simulink model "Test"  (R2023b)
settings: Solver=FixedStepDiscrete  StartTime=0.0  StopTime=inf  RelTol=1e-3
model workspace (MATLAB code in the model file):
  | cmdLim = Simulink.Parameter;
  | cmdLim.Value = 15;
  | cmdLim.Description = 'Limit for controlling the maximum surface command angle.';
  | cmdLim.Min = 0;
  | cmdLim.Max = 90;
  | cmdLim.DocUnits = 'deg';
  | 
  | dispGain = Simulink.Parameter;
  | dispGain.Value = 0.75;
  | dispGain.Description = 'Gain applied to the displacement error.';
  | dispGain.Min = 0;
  | dispGain.Max = [];
  | dispGain.DocUnits = 'deg/sec/deg';
  | 
  | dispLim = Simulink.Parameter;
  | dispLim.Value = 30;
  | dispLim.Description = 'Limit for controlling the maximum commanded angle.';
  | dispLim.Min = 0;
  | dispLim.Max = 180;
  | dispLim.DocUnits = 'deg';
  | 
  | intGain = Simulink.Parameter;
  | intGain.Value = 0.5;
  | intGain.Description = 'Gain applied to the integral error.';
  | intGain.Min = 0;
  | intGain.Max = [];
  | intGain.DocUnits = 'deg/sec/deg/sec';
  | 
  | intLim = Simulink.Parameter;
  | intLim.Value = 5;
  | intLim.Description = 'Limit for controlling the maximum commanded angle.';
  | intLim.Min = 0;
  | intLim.Max = 90;
  | intLim.DocUnits = 'deg';
  | 
  | rateGain = Simulink.Parameter;
  | rateGain.Value = 2;
  | rateGain.Description = 'Gain applied to the rate error.';
  | rateGain.Min = 0;
  | rateGain.Max = [];
  | rateGain.DocUnits = 'deg/deg/sec';
  | 
  | rateLim = Simulink.Parameter;
  | rateLim.Value = 6;
  | rateLim.Description = 'Limit for controlling the maximum commanded angle.';
  | rateLim.Min = 0;
  | rateLim.Max = 180;
  | rateLim.DocUnits = 'deg/sec';
  | 
  | hdgGain = Simulink.Parameter;
  | hdgGain.Value = 0.015;
libraries: simulink x33, arduinolib x17, hdlsllib x14, canmsglib x2
settings Model: RequirementInfo={} %GIDa_fe9045fd_0412_4b6e_8206_617cc20e6fde  DataDictionary=Time.sldd  FPTRunName=Active  ExtModeTrigDuration=2  Creator=jorda  LastModifiedBy=jorda
settings SolverCC: AlgebraicLoopSolver=TrustRegion  AutoInsertRateTranBlk=on
settings DataIOCC: SaveOutput=off  SignalLogging=off  DSMLogging=off  SaveTime=off
settings OptimizationCC: UseDivisionForNetSlopeComputation=on  GainParamInheritBuiltInType=on  UseFloatMulNetSlope=on  UseSpecifiedMinMax=on  EnhancedBackFolding=on  PassReuseOutputArgsAs=Individual arguments  ZeroExternalMemoryAtStartup=off  ZeroInternalMemoryAtStartup=off  NoFixptDivByZeroProtection=on  EfficientFloat2IntCast=on  LifeSpan=1  MaxStackSize=64  OptimizeBlockOrder=speed  DifferentSizesBufferReuse=on  OptimizationCustomize=off  EfficientTunableParamExpr=on
settings DebuggingCC: MultiTaskDSMMsg=none  UnconnectedInputMsg=warning  UnconnectedOutputMsg=warning  UnconnectedLineMsg=warning  SFUnexpectedBacktrackingDiag=warning  SFNoUnconditionalDefaultTransitionDiag=warning  SFExecutionAtInitializationDiag=none  ArithmeticOperatorsInVariantConditions=warning
settings HardwareCC: ProdBitPerInt=16  ProdBitPerPointer=16  ProdBitPerSizeT=16  ProdBitPerPtrDiffT=16  ProdLargestAtomicFloat=None  ProdWordSize=8  ProdHWDeviceType=Atmel->AVR
settings ModelReferenceCC: EnableRefExpFcnMdlSchedulingChecks=on
settings SFSimCC: MATLABDynamicMemAlloc=off
settings RTWCC: Description=Embedded Coder  SystemTargetFile=ert.tlc  HardwareBoard=Arduino Mega 2560  TemplateMakefile=ert_default_tmf  Toolchain=Arduino AVR  BuildConfiguration=Faster Runs  DLArmComputeVersion=19.05
settings CodeAppCC: ForceParamTrailComments=on  IgnoreCustomStorageClasses=off  OperatorAnnotations=on  SimulinkDataObjDesc=on  SFDataObjDesc=on  CustomSymbolStrGlobalVar=rt$N$M  CustomSymbolStrType=$N$M  CustomSymbolStrFcn=$N$M$F  CustomSymbolStrMacro=$N$M  InsertBlockDesc=on  EnableCustomComments=on  ReqsInCode=on
settings ERTTargetCC: UtilityFuncGeneration=Shared location  MultiwordLength=2048  IncludeMdlTerminateFcn=off  CombineSignalStateStructs=on  SuppressErrorStatus=on  SupportAbsoluteTime=off  SupportNonFinite=off  SupportComplex=off  SupportContinuousTime=on  SupportVariableSizeSignals=on  ExtModeTransport=3  ExtModeStaticAlloc=on  ExtModeAutomaticAllocSize=off  ExtModeStaticAllocSize=2048  ExtModeMexFile=ext_xcp  ExtModeIntrfLevel=Level2 - Open  ERTFilePackagingFormat=CompactWithDataFile
settings ConfigComp: CovScope=ReferencedModels  CovSaveName=covdata_rollAP  CovMetricSettings=dcmtrwe  CovHTMLOptions=-sRT=1 -aTS=1 -bRG=1 -bTC=1 -hTR=1 -nFC=0 -scm=1 -bcm=1 -xEv=0  CovSaveCumulativeToWorkspaceVar=on  CovSaveSingleToWorkspaceVar=on  CovCumulativeVarName=covCumulativeData_rollAP  CovReportOnPause=off  CovExternalEMLEnable=off  CovSFcnEnable=off

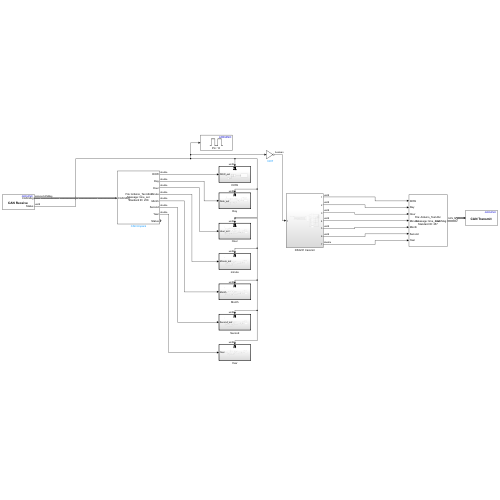
[thumbnail: Simulink's stored preview of the top-level diagram]
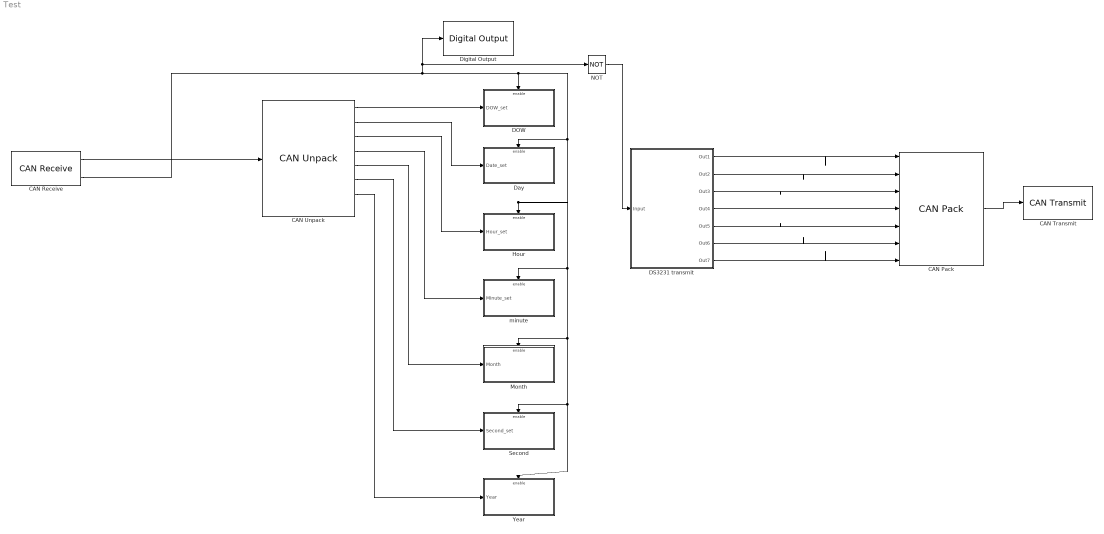
== system Test ==
  CAN Pack : canmsglib/CAN Pack  CANdbFile=C:\Users\jorda\Documents\Arduino_Test.dbc  MsgList=time_now  MsgName=time_now  MsgIDType=Standard (11-bit identifier)  MsgIdentifier=257  MsgLength=7  Remote=off  ApplyMinMax=off  BusOutput=on  SignalInfo={'DOW','37','3','LE','unsigned','Standard','0','1','0','0','7';'Day','24','5','LE','unsigned','Standard','0','1','0','0','31';'Hour','16','5','LE','unsigned','Standard','0','1','0','0','31';'Minute','8','6','LE','unsigned','Standard','0','1','0','0','63';'Month','32','4','LE','unsigned','Standard','0','1','0','0','15';'Second','0','6','LE','unsigned','Standard','0','1','0','0','63';'Year','40','12','LE','unsigned','Standard','0','1','0','0','4095'}
      settings: LibrarySourceBlock=embeddedtargetslib/Host Communication/CAN Pack  DataFormat=CANdb specified signals
  CAN Receive : arduinolib/CAN Receive  outputDataType=CAN Msg  identifierType=Standard (11-bit identifier)  messageId=100  msgLength=8  SampleTime=0.1  outputError=off  outputRemote=off
  CAN Transmit : arduinolib/CAN Transmit  inputDataType=CAN Msg  BlockingMode_=off  BlockTimeout_=1  outputStatus=off  identifierType=Standard (11-bit identifier)  messageId=102  msgLength=8  remoteFrame=off
  CAN Unpack : canmsglib/CAN Unpack  CANdbFile=C:\Users\jorda\Documents\Arduino_Test.dbc  MsgList=time_set  MsgName=time_set  MsgIDType=Standard (11-bit identifier)  MsgIdentifier=258  MsgLength=7  SignalInfo={'DOW','37','3','LE','unsigned','Standard','0','1','0','0','7';'Day','24','5','LE','unsigned','Standard','0','1','0','0','31';'Hour','16','5','LE','unsigned','Standard','0','1','0','0','31';'Minute','8','6','LE','unsigned','Standard','0','1','0','0','63';'Month','32','4','LE','unsigned','Standard','0','1','0','0','15';'Second','0','6','LE','unsigned','Standard','0','1','0','0','63';'Year','40','12','LE','unsigned','Standard','0','1','0','0','4095'}  IDPort=off  TimestampPort=off  ErrorPort=off  RemotePort=off  LengthPort=off  StatusPort=on  ApplyMinMax=off
      settings: LibrarySourceBlock=embeddedtargetslib/Host Communication/CAN Unpack  DataFormat=CANdb specified signals
  DOW : Subsystem
  DS3231 transmit : Subsystem
  Day : Subsystem
  Digital Output : arduinolib/Digital Output  pinNumber=13  Direction=output  blockPlatform=arduino
  Hour : Subsystem
  Month : Subsystem
  NOT : Logic  Operator=NOT  IconShape=distinctive  AllPortsSameDT=off  OutDataTypeStr=boolean
  Second : Subsystem
  Year : Subsystem
  minute : Subsystem
  wires:
  CAN Pack/1 -> CAN Transmit/1
  DS3231 transmit/1(Out1) -> CAN Pack/1
  DS3231 transmit/2(Out2) -> CAN Pack/2
  DS3231 transmit/3(Out3) -> CAN Pack/3
  DS3231 transmit/4(Out4) -> CAN Pack/4
  DS3231 transmit/5(Out5) -> CAN Pack/5
  DS3231 transmit/6(Out6) -> CAN Pack/6
  DS3231 transmit/7(Out7) -> CAN Pack/7
  CAN Receive/1 -> CAN Unpack/1
  CAN Receive/2 -> NOT/1, Digital Output/1, Day/Enable, Year/Enable, Second/Enable, Month/Enable, minute/Enable, Hour/Enable, DOW/Enable
  NOT/1 -> DS3231 transmit/1(Input)
  CAN Unpack/1 -> DOW/1(DOW_set)
  CAN Unpack/2 -> Day/1(Date_set)
  CAN Unpack/3 -> Hour/1(Hour_set)
  CAN Unpack/4 -> minute/1(Minute_set)
  CAN Unpack/5 -> Month/1(Month)
  CAN Unpack/6 -> Second/1(Second_set)
  CAN Unpack/7 -> Year/1(Year)

== system Test/DOW ==
  DOW_set : Inport
  Enable : EnablePort
  Bitwise AND : simulink/Logic and Bit Operations/Bitwise Operator  logicop=AND  UseBitMask=off  NumInputPorts=2  BitMask=bin2dec('11011001')  BitMaskRealWorld=Stored Integer
      settings: LibrarySourceBlock=|
      | simulink/Quick Insert/Logic and Bit
      | Operations/Bitwise AND
  Constant : Constant  Value=0x07
  Data Type Conversion : DataTypeConversion  OutDataTypeStr=uint8  SaturateOnIntegerOverflow=off  RndMeth=Floor
  I2C Write : arduinolib/I2C Write  I2CModule=0  Mode=Master  SlaveAddress=0x68  SlaveByteOrder=BigEndian  Direction=Transmitter  RegisterAddressMode=on  RegisterAddress=0x03  SlaveDataType=uint8  DataLength=1  NoAck=off  RepeatedStart=off  OutputStatus=off  blockPlatform=ARDUINO
  wires:
  Bitwise AND/1 -> I2C Write/1
  DOW_set/1 -> Data Type Conversion/1
  Constant/1 -> Bitwise AND/2
  Data Type Conversion/1 -> Bitwise AND/1

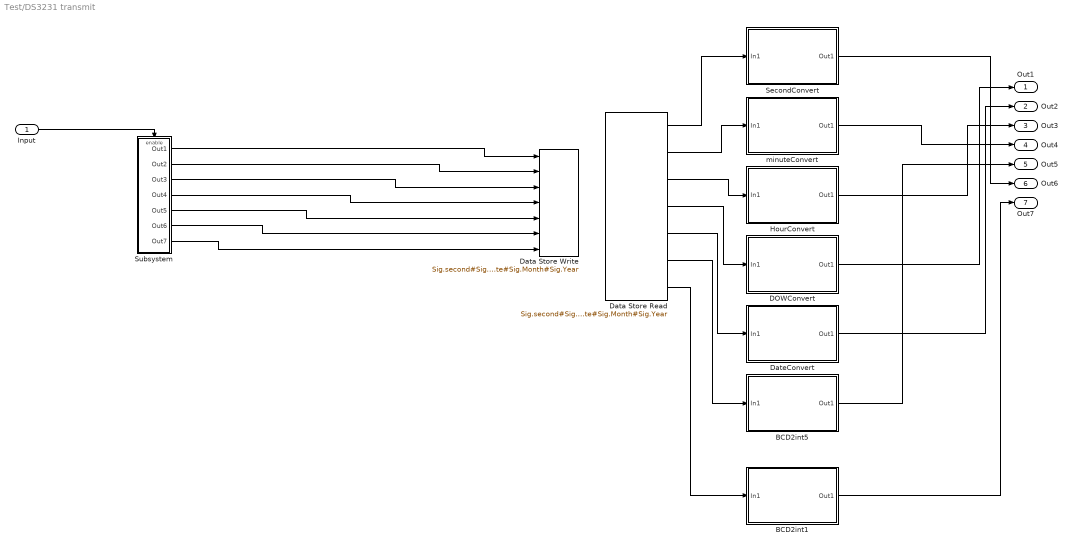
== system Test/DS3231 transmit ==
  Input : Inport
  BCD2int1 : Subsystem
  BCD2int5 : Subsystem
  DOWConvert : Subsystem
  Data Store Read : DataStoreRead  DataStoreName=Sig  DataStoreElements=Sig.second#Sig.minute#Sig.hour#Sig.DOW#Sig.Date#Sig.Month#Sig.Year  IndexOptions=Index vector (dialog)  Indices=1  OutputSizes=1
  Data Store Write : DataStoreWrite  DataStoreName=Sig  DataStoreElements=Sig.second#Sig.minute#Sig.hour#Sig.DOW#Sig.Date#Sig.Month#Sig.Year  IndexOptions=Index vector (dialog)  Indices=1  OutputSizes=1
  DateConvert : Subsystem
  HourConvert : Subsystem
  SecondConvert : Subsystem
  Subsystem : Subsystem
  minuteConvert : Subsystem
  Out1 : Outport
  Out2 : Outport  Port=2
  Out3 : Outport  Port=3
  Out4 : Outport  Port=4
  Out5 : Outport  Port=5
  Out6 : Outport  Port=6
  Out7 : Outport  Port=7
  wires:
  Data Store Read/6 -> BCD2int5/1(In1)
  Data Store Read/3 -> HourConvert/1(In1)
  Data Store Read/1 -> SecondConvert/1(In1)
  SecondConvert/1(Out1) -> Out6/1
  Data Store Read/7 -> BCD2int1/1(In1)
  Data Store Read/2 -> minuteConvert/1(In1)
  Data Store Read/4 -> DOWConvert/1(In1)
  Data Store Read/5 -> DateConvert/1(In1)
  HourConvert/1(Out1) -> Out3/1
  DateConvert/1(Out1) -> Out2/1
  DOWConvert/1(Out1) -> Out1/1
  BCD2int5/1(Out1) -> Out5/1
  minuteConvert/1(Out1) -> Out4/1
  BCD2int1/1(Out1) -> Out7/1
  Subsystem/1(Out1) -> Data Store Write/1
  Subsystem/2(Out2) -> Data Store Write/2
  Subsystem/3(Out3) -> Data Store Write/3
  Subsystem/4(Out4) -> Data Store Write/4
  Subsystem/5(Out5) -> Data Store Write/5
  Subsystem/6(Out6) -> Data Store Write/6
  Subsystem/7(Out7) -> Data Store Write/7
  Input/1 -> Subsystem/Enable

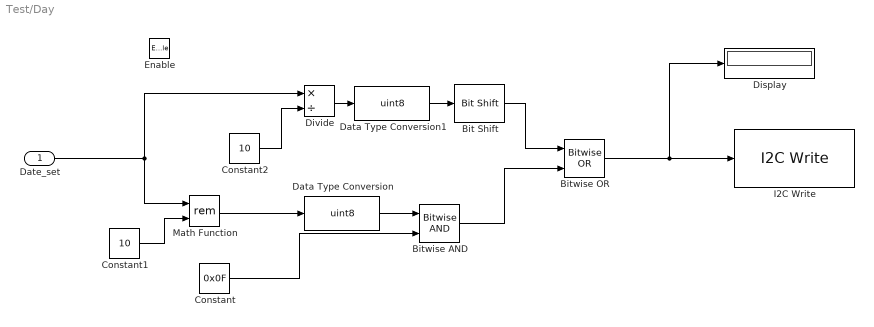
== system Test/Day ==
  Date_set : Inport
  Enable : EnablePort
  Bit Shift : hdlsllib/Logic and Bit Operations/Bit Shift  mode=Shift Left Logical  N=4
  Bitwise AND : simulink/Logic and Bit Operations/Bitwise Operator  logicop=AND  UseBitMask=off  NumInputPorts=2  BitMask=bin2dec('11011001')  BitMaskRealWorld=Stored Integer
      settings: LibrarySourceBlock=|
      | simulink/Quick Insert/Logic and Bit
      | Operations/Bitwise AND
  Bitwise OR : simulink/Logic and Bit Operations/Bitwise Operator  logicop=OR  UseBitMask=off  NumInputPorts=2  BitMask=bin2dec('11011001')  BitMaskRealWorld=Stored Integer
      settings: LibrarySourceBlock=|
      | simulink/Quick Insert/Logic and Bit
      | Operations/Bitwise OR
  Constant : Constant  Value=0x0F
  Constant1 : Constant  Value=10
  Constant2 : Constant  Value=10
  Data Type Conversion : DataTypeConversion  OutDataTypeStr=uint8  SaturateOnIntegerOverflow=off  RndMeth=Floor
  Data Type Conversion1 : DataTypeConversion  OutDataTypeStr=uint8  SaturateOnIntegerOverflow=off  RndMeth=Floor
  Display : Display
      settings: Format=hex (Stored Integer)
  Divide : Product  Inputs=*/
  I2C Write : arduinolib/I2C Write  I2CModule=0  Mode=Master  SlaveAddress=0x68  SlaveByteOrder=BigEndian  Direction=Transmitter  RegisterAddressMode=on  RegisterAddress=0x04  SlaveDataType=uint8  DataLength=1  NoAck=off  RepeatedStart=off  OutputStatus=off  blockPlatform=ARDUINO
  Math Function : Math  Operator=rem
  wires:
  Constant/1 -> Bitwise AND/2
  Constant2/1 -> Divide/2
  Bit Shift/1 -> Bitwise OR/1
  Bitwise AND/1 -> Bitwise OR/2
  Data Type Conversion1/1 -> Bit Shift/1
  Divide/1 -> Data Type Conversion1/1
  Bitwise OR/1 -> Display/1, I2C Write/1
  Data Type Conversion/1 -> Bitwise AND/1
  Constant1/1 -> Math Function/2
  Math Function/1 -> Data Type Conversion/1
  Date_set/1 -> Math Function/1, Divide/1

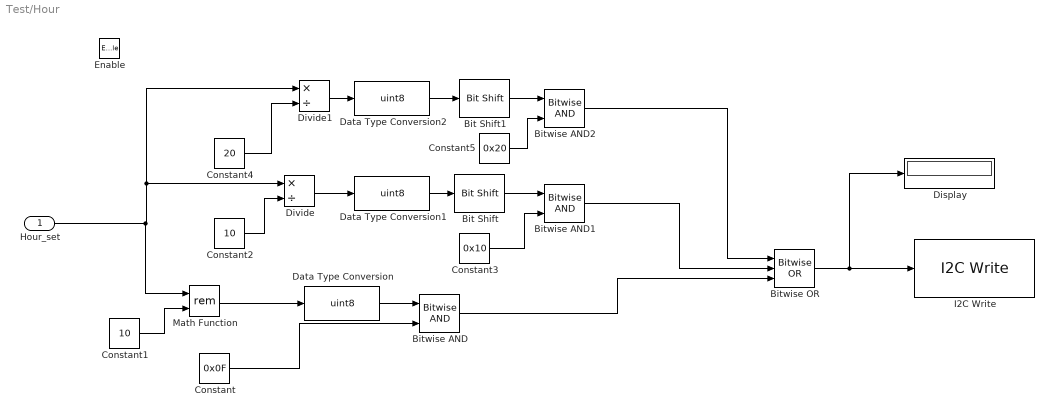
== system Test/Hour ==
  Hour_set : Inport
  Enable : EnablePort
  Bit Shift : hdlsllib/Logic and Bit Operations/Bit Shift  mode=Shift Left Logical  N=4
  Bit Shift1 : hdlsllib/Logic and Bit Operations/Bit Shift  mode=Shift Left Logical  N=5
  Bitwise AND : simulink/Logic and Bit Operations/Bitwise Operator  logicop=AND  UseBitMask=off  NumInputPorts=2  BitMask=bin2dec('11011001')  BitMaskRealWorld=Stored Integer
      settings: LibrarySourceBlock=|
      | simulink/Quick Insert/Logic and Bit
      | Operations/Bitwise AND
  Bitwise AND1 : simulink/Logic and Bit Operations/Bitwise Operator  logicop=AND  UseBitMask=off  NumInputPorts=2  BitMask=bin2dec('11011001')  BitMaskRealWorld=Stored Integer
      settings: LibrarySourceBlock=|
      | simulink/Quick Insert/Logic and Bit
      | Operations/Bitwise AND
  Bitwise AND2 : simulink/Logic and Bit Operations/Bitwise Operator  logicop=AND  UseBitMask=off  NumInputPorts=2  BitMask=bin2dec('11011001')  BitMaskRealWorld=Stored Integer
      settings: LibrarySourceBlock=|
      | simulink/Quick Insert/Logic and Bit
      | Operations/Bitwise AND
  Bitwise OR : simulink/Logic and Bit Operations/Bitwise Operator  logicop=OR  UseBitMask=off  NumInputPorts=3  BitMask=bin2dec('11011001')  BitMaskRealWorld=Stored Integer
      settings: LibrarySourceBlock=|
      | simulink/Quick Insert/Logic and Bit
      | Operations/Bitwise OR
  Constant : Constant  Value=0x0F
  Constant1 : Constant  Value=10
  Constant2 : Constant  Value=10
  Constant3 : Constant  Value=0x10
  Constant4 : Constant  Value=20
  Constant5 : Constant  Value=0x20
  Data Type Conversion : DataTypeConversion  OutDataTypeStr=uint8  SaturateOnIntegerOverflow=off  RndMeth=Floor
  Data Type Conversion1 : DataTypeConversion  OutDataTypeStr=uint8  SaturateOnIntegerOverflow=off  RndMeth=Floor
  Data Type Conversion2 : DataTypeConversion  OutDataTypeStr=uint8  SaturateOnIntegerOverflow=off  RndMeth=Floor
  Display : Display
      settings: Format=hex (Stored Integer)
  Divide : Product  Inputs=*/
  Divide1 : Product  Inputs=*/
  I2C Write : arduinolib/I2C Write  I2CModule=0  Mode=Master  SlaveAddress=0x68  SlaveByteOrder=BigEndian  Direction=Transmitter  RegisterAddressMode=on  RegisterAddress=0x02  SlaveDataType=uint8  DataLength=1  NoAck=off  RepeatedStart=off  OutputStatus=off  blockPlatform=ARDUINO
  Math Function : Math  Operator=rem
  wires:
  Constant/1 -> Bitwise AND/2
  Constant2/1 -> Divide/2
  Bitwise AND/1 -> Bitwise OR/3
  Data Type Conversion1/1 -> Bit Shift/1
  Divide/1 -> Data Type Conversion1/1
  Bitwise OR/1 -> Display/1, I2C Write/1
  Data Type Conversion/1 -> Bitwise AND/1
  Constant1/1 -> Math Function/2
  Math Function/1 -> Data Type Conversion/1
  Bit Shift/1 -> Bitwise AND1/1
  Constant3/1 -> Bitwise AND1/2
  Bitwise AND1/1 -> Bitwise OR/2
  Divide1/1 -> Data Type Conversion2/1
  Constant4/1 -> Divide1/2
  Data Type Conversion2/1 -> Bit Shift1/1
  Bit Shift1/1 -> Bitwise AND2/1
  Constant5/1 -> Bitwise AND2/2
  Bitwise AND2/1 -> Bitwise OR/1
  Hour_set/1 -> Math Function/1, Divide/1, Divide1/1

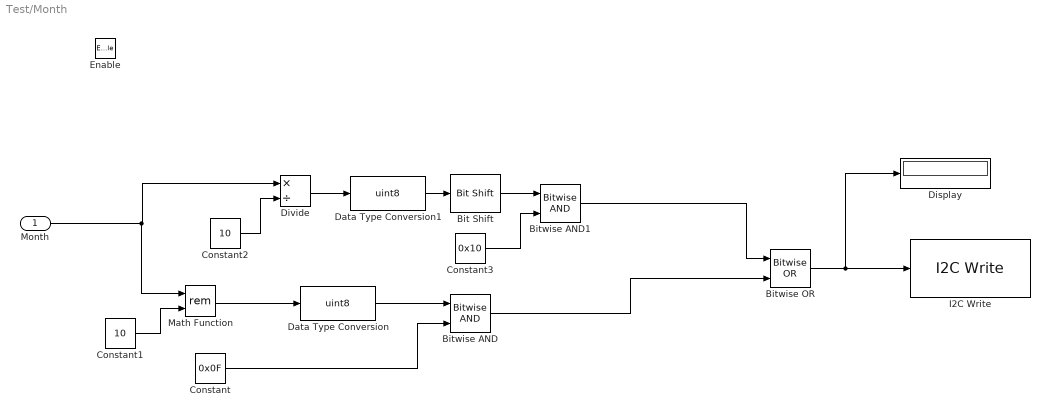
== system Test/Month ==
  Month : Inport
  Enable : EnablePort
  Bit Shift : hdlsllib/Logic and Bit Operations/Bit Shift  mode=Shift Left Logical  N=4
  Bitwise AND : simulink/Logic and Bit Operations/Bitwise Operator  logicop=AND  UseBitMask=off  NumInputPorts=2  BitMask=bin2dec('11011001')  BitMaskRealWorld=Stored Integer
      settings: LibrarySourceBlock=|
      | simulink/Quick Insert/Logic and Bit
      | Operations/Bitwise AND
  Bitwise AND1 : simulink/Logic and Bit Operations/Bitwise Operator  logicop=AND  UseBitMask=off  NumInputPorts=2  BitMask=bin2dec('11011001')  BitMaskRealWorld=Stored Integer
      settings: LibrarySourceBlock=|
      | simulink/Quick Insert/Logic and Bit
      | Operations/Bitwise AND
  Bitwise OR : simulink/Logic and Bit Operations/Bitwise Operator  logicop=OR  UseBitMask=off  NumInputPorts=2  BitMask=bin2dec('11011001')  BitMaskRealWorld=Stored Integer
      settings: LibrarySourceBlock=|
      | simulink/Quick Insert/Logic and Bit
      | Operations/Bitwise OR
  Constant : Constant  Value=0x0F
  Constant1 : Constant  Value=10
  Constant2 : Constant  Value=10
  Constant3 : Constant  Value=0x10
  Data Type Conversion : DataTypeConversion  OutDataTypeStr=uint8  SaturateOnIntegerOverflow=off  RndMeth=Floor
  Data Type Conversion1 : DataTypeConversion  OutDataTypeStr=uint8  SaturateOnIntegerOverflow=off  RndMeth=Floor
  Display : Display
      settings: Format=hex (Stored Integer)
  Divide : Product  Inputs=*/
  I2C Write : arduinolib/I2C Write  I2CModule=0  Mode=Master  SlaveAddress=0x68  SlaveByteOrder=BigEndian  Direction=Transmitter  RegisterAddressMode=on  RegisterAddress=0x05  SlaveDataType=uint8  DataLength=1  NoAck=off  RepeatedStart=off  OutputStatus=off  blockPlatform=ARDUINO
  Math Function : Math  Operator=rem
  wires:
  Constant/1 -> Bitwise AND/2
  Constant2/1 -> Divide/2
  Bitwise AND/1 -> Bitwise OR/2
  Data Type Conversion1/1 -> Bit Shift/1
  Divide/1 -> Data Type Conversion1/1
  Bitwise OR/1 -> Display/1, I2C Write/1
  Data Type Conversion/1 -> Bitwise AND/1
  Constant1/1 -> Math Function/2
  Math Function/1 -> Data Type Conversion/1
  Bit Shift/1 -> Bitwise AND1/1
  Constant3/1 -> Bitwise AND1/2
  Bitwise AND1/1 -> Bitwise OR/1
  Month/1 -> Math Function/1, Divide/1

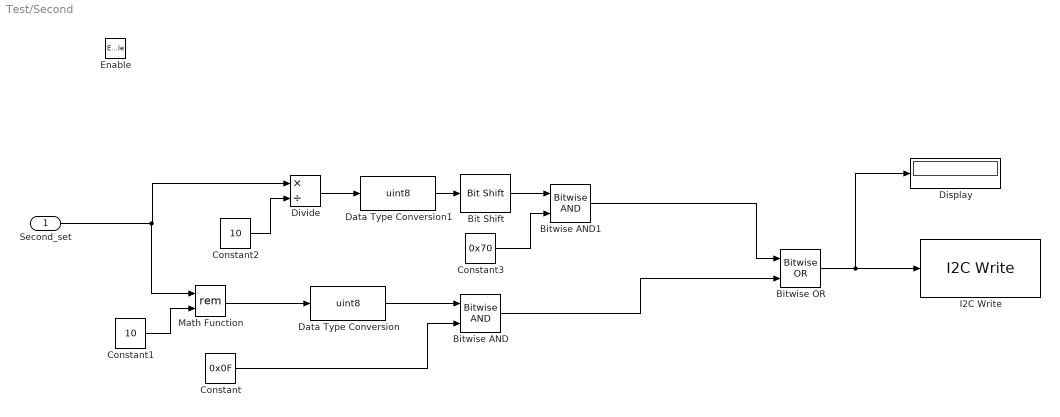
== system Test/Second ==
  Second_set : Inport
  Enable : EnablePort
  Bit Shift : hdlsllib/Logic and Bit Operations/Bit Shift  mode=Shift Left Logical  N=4
  Bitwise AND : simulink/Logic and Bit Operations/Bitwise Operator  logicop=AND  UseBitMask=off  NumInputPorts=2  BitMask=bin2dec('11011001')  BitMaskRealWorld=Stored Integer
      settings: LibrarySourceBlock=|
      | simulink/Quick Insert/Logic and Bit
      | Operations/Bitwise AND
  Bitwise AND1 : simulink/Logic and Bit Operations/Bitwise Operator  logicop=AND  UseBitMask=off  NumInputPorts=2  BitMask=bin2dec('11011001')  BitMaskRealWorld=Stored Integer
      settings: LibrarySourceBlock=|
      | simulink/Quick Insert/Logic and Bit
      | Operations/Bitwise AND
  Bitwise OR : simulink/Logic and Bit Operations/Bitwise Operator  logicop=OR  UseBitMask=off  NumInputPorts=2  BitMask=bin2dec('11011001')  BitMaskRealWorld=Stored Integer
      settings: LibrarySourceBlock=|
      | simulink/Quick Insert/Logic and Bit
      | Operations/Bitwise OR
  Constant : Constant  Value=0x0F
  Constant1 : Constant  Value=10
  Constant2 : Constant  Value=10
  Constant3 : Constant  Value=0x70
  Data Type Conversion : DataTypeConversion  OutDataTypeStr=uint8  SaturateOnIntegerOverflow=off  RndMeth=Floor
  Data Type Conversion1 : DataTypeConversion  OutDataTypeStr=uint8  SaturateOnIntegerOverflow=off  RndMeth=Floor
  Display : Display
      settings: Format=hex (Stored Integer)
  Divide : Product  Inputs=*/
  I2C Write : arduinolib/I2C Write  I2CModule=0  Mode=Master  SlaveAddress=0x68  SlaveByteOrder=BigEndian  Direction=Transmitter  RegisterAddressMode=on  RegisterAddress=0x00  SlaveDataType=uint8  DataLength=1  NoAck=off  RepeatedStart=off  OutputStatus=off  blockPlatform=ARDUINO
  Math Function : Math  Operator=rem
  wires:
  Constant/1 -> Bitwise AND/2
  Constant2/1 -> Divide/2
  Bitwise AND/1 -> Bitwise OR/2
  Data Type Conversion1/1 -> Bit Shift/1
  Divide/1 -> Data Type Conversion1/1
  Bitwise OR/1 -> Display/1, I2C Write/1
  Data Type Conversion/1 -> Bitwise AND/1
  Constant1/1 -> Math Function/2
  Math Function/1 -> Data Type Conversion/1
  Bit Shift/1 -> Bitwise AND1/1
  Constant3/1 -> Bitwise AND1/2
  Bitwise AND1/1 -> Bitwise OR/1
  Second_set/1 -> Math Function/1, Divide/1

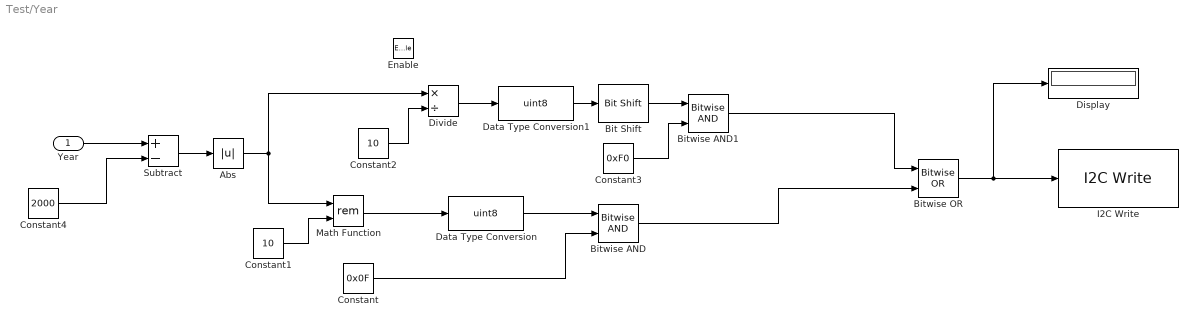
== system Test/Year ==
  Year : Inport
  Enable : EnablePort
  Abs : Abs  SaturateOnIntegerOverflow=off
  Bit Shift : hdlsllib/Logic and Bit Operations/Bit Shift  mode=Shift Left Logical  N=4
  Bitwise AND : simulink/Logic and Bit Operations/Bitwise Operator  logicop=AND  UseBitMask=off  NumInputPorts=2  BitMask=bin2dec('11011001')  BitMaskRealWorld=Stored Integer
      settings: LibrarySourceBlock=|
      | simulink/Quick Insert/Logic and Bit
      | Operations/Bitwise AND
  Bitwise AND1 : simulink/Logic and Bit Operations/Bitwise Operator  logicop=AND  UseBitMask=off  NumInputPorts=2  BitMask=bin2dec('11011001')  BitMaskRealWorld=Stored Integer
      settings: LibrarySourceBlock=|
      | simulink/Quick Insert/Logic and Bit
      | Operations/Bitwise AND
  Bitwise OR : simulink/Logic and Bit Operations/Bitwise Operator  logicop=OR  UseBitMask=off  NumInputPorts=2  BitMask=bin2dec('11011001')  BitMaskRealWorld=Stored Integer
      settings: LibrarySourceBlock=|
      | simulink/Quick Insert/Logic and Bit
      | Operations/Bitwise OR
  Constant : Constant  Value=0x0F
  Constant1 : Constant  Value=10
  Constant2 : Constant  Value=10
  Constant3 : Constant  Value=0xF0
  Constant4 : Constant  Value=2000
  Data Type Conversion : DataTypeConversion  OutDataTypeStr=uint8  SaturateOnIntegerOverflow=off  RndMeth=Floor
  Data Type Conversion1 : DataTypeConversion  OutDataTypeStr=uint8  SaturateOnIntegerOverflow=off  RndMeth=Floor
  Display : Display
      settings: Format=hex (Stored Integer)
  Divide : Product  Inputs=*/
  I2C Write : arduinolib/I2C Write  I2CModule=0  Mode=Master  SlaveAddress=0x68  SlaveByteOrder=BigEndian  Direction=Transmitter  RegisterAddressMode=on  RegisterAddress=0x06  SlaveDataType=uint8  DataLength=1  NoAck=off  RepeatedStart=off  OutputStatus=off  blockPlatform=ARDUINO
  Math Function : Math  Operator=rem
  Subtract : Sum  Inputs=+-
  wires:
  Constant/1 -> Bitwise AND/2
  Constant2/1 -> Divide/2
  Bitwise AND/1 -> Bitwise OR/2
  Data Type Conversion1/1 -> Bit Shift/1
  Divide/1 -> Data Type Conversion1/1
  Bitwise OR/1 -> Display/1, I2C Write/1
  Data Type Conversion/1 -> Bitwise AND/1
  Constant1/1 -> Math Function/2
  Math Function/1 -> Data Type Conversion/1
  Bit Shift/1 -> Bitwise AND1/1
  Constant3/1 -> Bitwise AND1/2
  Bitwise AND1/1 -> Bitwise OR/1
  Constant4/1 -> Subtract/2
  Subtract/1 -> Abs/1
  Year/1 -> Subtract/1
  Abs/1 -> Math Function/1, Divide/1

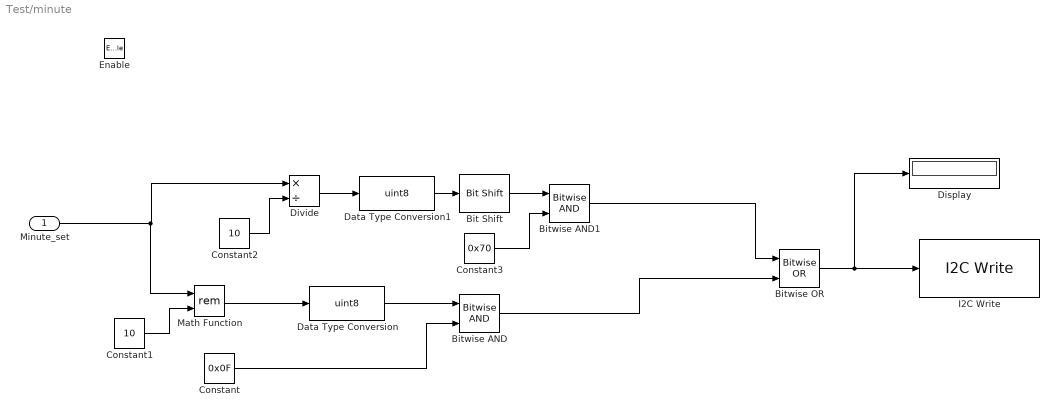
== system Test/minute ==
  Minute_set : Inport
  Enable : EnablePort
  Bit Shift : hdlsllib/Logic and Bit Operations/Bit Shift  mode=Shift Left Logical  N=4
  Bitwise AND : simulink/Logic and Bit Operations/Bitwise Operator  logicop=AND  UseBitMask=off  NumInputPorts=2  BitMask=bin2dec('11011001')  BitMaskRealWorld=Stored Integer
      settings: LibrarySourceBlock=|
      | simulink/Quick Insert/Logic and Bit
      | Operations/Bitwise AND
  Bitwise AND1 : simulink/Logic and Bit Operations/Bitwise Operator  logicop=AND  UseBitMask=off  NumInputPorts=2  BitMask=bin2dec('11011001')  BitMaskRealWorld=Stored Integer
      settings: LibrarySourceBlock=|
      | simulink/Quick Insert/Logic and Bit
      | Operations/Bitwise AND
  Bitwise OR : simulink/Logic and Bit Operations/Bitwise Operator  logicop=OR  UseBitMask=off  NumInputPorts=2  BitMask=bin2dec('11011001')  BitMaskRealWorld=Stored Integer
      settings: LibrarySourceBlock=|
      | simulink/Quick Insert/Logic and Bit
      | Operations/Bitwise OR
  Constant : Constant  Value=0x0F
  Constant1 : Constant  Value=10
  Constant2 : Constant  Value=10
  Constant3 : Constant  Value=0x70
  Data Type Conversion : DataTypeConversion  OutDataTypeStr=uint8  SaturateOnIntegerOverflow=off  RndMeth=Floor
  Data Type Conversion1 : DataTypeConversion  OutDataTypeStr=uint8  SaturateOnIntegerOverflow=off  RndMeth=Floor
  Display : Display
      settings: Format=hex (Stored Integer)
  Divide : Product  Inputs=*/
  I2C Write : arduinolib/I2C Write  I2CModule=0  Mode=Master  SlaveAddress=0x68  SlaveByteOrder=BigEndian  Direction=Transmitter  RegisterAddressMode=on  RegisterAddress=0x01  SlaveDataType=uint8  DataLength=1  NoAck=off  RepeatedStart=off  OutputStatus=off  blockPlatform=ARDUINO
  Math Function : Math  Operator=rem
  wires:
  Constant/1 -> Bitwise AND/2
  Constant2/1 -> Divide/2
  Bitwise AND/1 -> Bitwise OR/2
  Data Type Conversion1/1 -> Bit Shift/1
  Divide/1 -> Data Type Conversion1/1
  Bitwise OR/1 -> Display/1, I2C Write/1
  Data Type Conversion/1 -> Bitwise AND/1
  Constant1/1 -> Math Function/2
  Math Function/1 -> Data Type Conversion/1
  Bit Shift/1 -> Bitwise AND1/1
  Constant3/1 -> Bitwise AND1/2
  Bitwise AND1/1 -> Bitwise OR/1
  Minute_set/1 -> Math Function/1, Divide/1

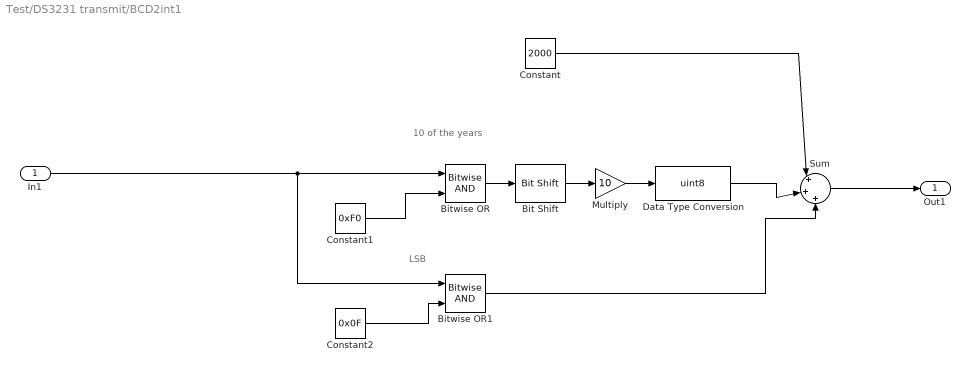
== system Test/DS3231 transmit/BCD2int1 ==
  note: LSB
  note: 10 of the years
  In1 : Inport
  Bit Shift : hdlsllib/Logic and Bit Operations/Bit Shift  mode=Shift Right Logical  N=4
  Bitwise OR : simulink/Logic and Bit Operations/Bitwise Operator  logicop=AND  UseBitMask=off  NumInputPorts=2  BitMask=bin2dec('0000FFFF')  BitMaskRealWorld=Stored Integer
      settings: LibrarySourceBlock=|
      | simulink/Quick Insert/Logic and Bit
      | Operations/Bitwise OR
  Bitwise OR1 : simulink/Logic and Bit Operations/Bitwise Operator  logicop=AND  UseBitMask=off  NumInputPorts=2  BitMask=bin2dec('0000FFFF')  BitMaskRealWorld=Stored Integer
      settings: LibrarySourceBlock=|
      | simulink/Quick Insert/Logic and Bit
      | Operations/Bitwise OR
  Constant : Constant  Value=2000
  Constant1 : Constant  Value=0xF0
  Constant2 : Constant  Value=0x0F
  Data Type Conversion : DataTypeConversion  OutDataTypeStr=uint8  SaturateOnIntegerOverflow=off  RndMeth=Floor
  Multiply : Gain  Gain=10  ParamDataTypeStr=Inherit: Same as input  LockScale=on
  Sum : Sum  Inputs=|+|+|+
  Out1 : Outport
  wires:
  Bitwise OR1/1 -> Sum/3
  Constant1/1 -> Bitwise OR/2
  Bit Shift/1 -> Multiply/1
  Bitwise OR/1 -> Bit Shift/1
  Data Type Conversion/1 -> Sum/2
  Multiply/1 -> Data Type Conversion/1
  Constant2/1 -> Bitwise OR1/2
  Sum/1 -> Out1/1
  In1/1 -> Bitwise OR1/1, Bitwise OR/1
  Constant/1 -> Sum/1

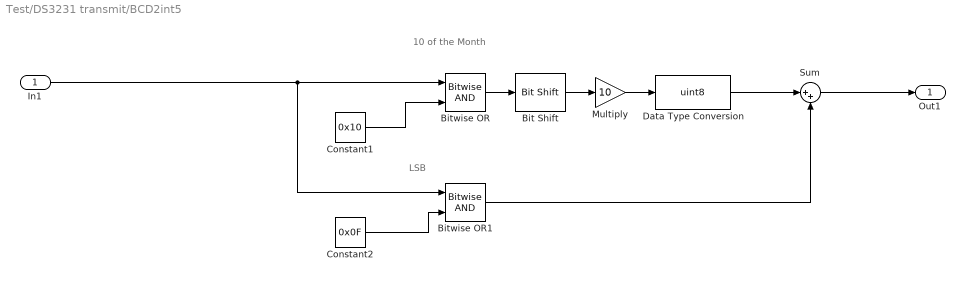
== system Test/DS3231 transmit/BCD2int5 ==
  note: LSB
  note: 10 of the Month
  In1 : Inport
  Bit Shift : hdlsllib/Logic and Bit Operations/Bit Shift  mode=Shift Right Logical  N=4
  Bitwise OR : simulink/Logic and Bit Operations/Bitwise Operator  logicop=AND  UseBitMask=off  NumInputPorts=2  BitMask=bin2dec('0000FFFF')  BitMaskRealWorld=Stored Integer
      settings: LibrarySourceBlock=|
      | simulink/Quick Insert/Logic and Bit
      | Operations/Bitwise OR
  Bitwise OR1 : simulink/Logic and Bit Operations/Bitwise Operator  logicop=AND  UseBitMask=off  NumInputPorts=2  BitMask=bin2dec('0000FFFF')  BitMaskRealWorld=Stored Integer
      settings: LibrarySourceBlock=|
      | simulink/Quick Insert/Logic and Bit
      | Operations/Bitwise OR
  Constant1 : Constant  Value=0x10
  Constant2 : Constant  Value=0x0F
  Data Type Conversion : DataTypeConversion  OutDataTypeStr=uint8  SaturateOnIntegerOverflow=off  RndMeth=Floor
  Multiply : Gain  Gain=10  ParamDataTypeStr=Inherit: Same as input  LockScale=on
  Sum : Sum  Inputs=|++
  Out1 : Outport
  wires:
  Bitwise OR1/1 -> Sum/2
  Constant1/1 -> Bitwise OR/2
  Bit Shift/1 -> Multiply/1
  Bitwise OR/1 -> Bit Shift/1
  Data Type Conversion/1 -> Sum/1
  Multiply/1 -> Data Type Conversion/1
  Constant2/1 -> Bitwise OR1/2
  Sum/1 -> Out1/1
  In1/1 -> Bitwise OR1/1, Bitwise OR/1

== system Test/DS3231 transmit/DOWConvert ==
  In1 : Inport
  Bitwise OR1 : simulink/Logic and Bit Operations/Bitwise Operator  logicop=AND  UseBitMask=off  NumInputPorts=2  BitMask=bin2dec('0000FFFF')  BitMaskRealWorld=Stored Integer
      settings: LibrarySourceBlock=|
      | simulink/Quick Insert/Logic and Bit
      | Operations/Bitwise OR
  Constant2 : Constant  Value=0x0F
  Out1 : Outport
  wires:
  Constant2/1 -> Bitwise OR1/2
  Bitwise OR1/1 -> Out1/1
  In1/1 -> Bitwise OR1/1

== system Test/DS3231 transmit/DateConvert ==
  note: LSB
  note: The 10th of Date
  In1 : Inport
  Bit Shift : hdlsllib/Logic and Bit Operations/Bit Shift  mode=Shift Right Logical  N=4
  Bitwise OR : simulink/Logic and Bit Operations/Bitwise Operator  logicop=AND  UseBitMask=off  NumInputPorts=2  BitMask=bin2dec('0000FFFF')  BitMaskRealWorld=Stored Integer
      settings: LibrarySourceBlock=|
      | simulink/Quick Insert/Logic and Bit
      | Operations/Bitwise OR
  Bitwise OR1 : simulink/Logic and Bit Operations/Bitwise Operator  logicop=AND  UseBitMask=off  NumInputPorts=2  BitMask=bin2dec('0000FFFF')  BitMaskRealWorld=Stored Integer
      settings: LibrarySourceBlock=|
      | simulink/Quick Insert/Logic and Bit
      | Operations/Bitwise OR
  Constant1 : Constant  Value=0x30
  Constant2 : Constant  Value=0x0F
  Data Type Conversion : DataTypeConversion  OutDataTypeStr=uint8  SaturateOnIntegerOverflow=off  RndMeth=Floor
  Multiply : Gain  Gain=10  ParamDataTypeStr=Inherit: Same as input  LockScale=on
  Sum : Sum  Inputs=|++
  Out1 : Outport
  wires:
  Bitwise OR1/1 -> Sum/2
  Constant1/1 -> Bitwise OR/2
  Bit Shift/1 -> Multiply/1
  Bitwise OR/1 -> Bit Shift/1
  Data Type Conversion/1 -> Sum/1
  Multiply/1 -> Data Type Conversion/1
  Constant2/1 -> Bitwise OR1/2
  Sum/1 -> Out1/1
  In1/1 -> Bitwise OR1/1, Bitwise OR/1

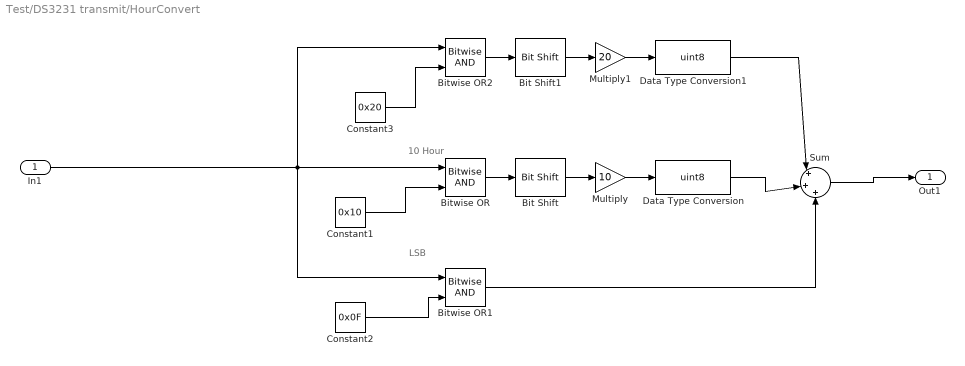
== system Test/DS3231 transmit/HourConvert ==
  note: LSB
  note: 10 Hour
  In1 : Inport
  Bit Shift : hdlsllib/Logic and Bit Operations/Bit Shift  mode=Shift Right Logical  N=4
  Bit Shift1 : hdlsllib/Logic and Bit Operations/Bit Shift  mode=Shift Right Logical  N=5
  Bitwise OR : simulink/Logic and Bit Operations/Bitwise Operator  logicop=AND  UseBitMask=off  NumInputPorts=2  BitMask=bin2dec('0000FFFF')  BitMaskRealWorld=Stored Integer
      settings: LibrarySourceBlock=|
      | simulink/Quick Insert/Logic and Bit
      | Operations/Bitwise OR
  Bitwise OR1 : simulink/Logic and Bit Operations/Bitwise Operator  logicop=AND  UseBitMask=off  NumInputPorts=2  BitMask=bin2dec('0000FFFF')  BitMaskRealWorld=Stored Integer
      settings: LibrarySourceBlock=|
      | simulink/Quick Insert/Logic and Bit
      | Operations/Bitwise OR
  Bitwise OR2 : simulink/Logic and Bit Operations/Bitwise Operator  logicop=AND  UseBitMask=off  NumInputPorts=2  BitMask=bin2dec('0000FFFF')  BitMaskRealWorld=Stored Integer
      settings: LibrarySourceBlock=|
      | simulink/Quick Insert/Logic and Bit
      | Operations/Bitwise OR
  Constant1 : Constant  Value=0x10
  Constant2 : Constant  Value=0x0F
  Constant3 : Constant  Value=0x20
  Data Type Conversion : DataTypeConversion  OutDataTypeStr=uint8  SaturateOnIntegerOverflow=off  RndMeth=Floor
  Data Type Conversion1 : DataTypeConversion  OutDataTypeStr=uint8  SaturateOnIntegerOverflow=off  RndMeth=Floor
  Multiply : Gain  Gain=10  ParamDataTypeStr=Inherit: Same as input  LockScale=on
  Multiply1 : Gain  Gain=20  ParamDataTypeStr=Inherit: Same as input  LockScale=on
  Sum : Sum  Inputs=|+|+|+
  Out1 : Outport
  wires:
  Constant1/1 -> Bitwise OR/2
  Bit Shift/1 -> Multiply/1
  Bitwise OR/1 -> Bit Shift/1
  Multiply/1 -> Data Type Conversion/1
  Constant2/1 -> Bitwise OR1/2
  Sum/1 -> Out1/1
  In1/1 -> Bitwise OR2/1, Bitwise OR1/1, Bitwise OR/1
  Bitwise OR2/1 -> Bit Shift1/1
  Bit Shift1/1 -> Multiply1/1
  Multiply1/1 -> Data Type Conversion1/1
  Bitwise OR1/1 -> Sum/3
  Data Type Conversion/1 -> Sum/2
  Data Type Conversion1/1 -> Sum/1
  Constant3/1 -> Bitwise OR2/2

== system Test/DS3231 transmit/SecondConvert ==
  note: LSB
  note: MSB
  In1 : Inport
  Bit Shift : hdlsllib/Logic and Bit Operations/Bit Shift  mode=Shift Right Logical  N=4
  Bitwise OR : simulink/Logic and Bit Operations/Bitwise Operator  logicop=AND  UseBitMask=off  NumInputPorts=2  BitMask=bin2dec('0000FFFF')  BitMaskRealWorld=Stored Integer
      settings: LibrarySourceBlock=|
      | simulink/Quick Insert/Logic and Bit
      | Operations/Bitwise OR
  Bitwise OR1 : simulink/Logic and Bit Operations/Bitwise Operator  logicop=AND  UseBitMask=off  NumInputPorts=2  BitMask=bin2dec('0000FFFF')  BitMaskRealWorld=Stored Integer
      settings: LibrarySourceBlock=|
      | simulink/Quick Insert/Logic and Bit
      | Operations/Bitwise OR
  Constant1 : Constant  Value=0xF0
  Constant2 : Constant  Value=0x0F
  Data Type Conversion : DataTypeConversion  OutDataTypeStr=uint8  SaturateOnIntegerOverflow=off  RndMeth=Floor
  Multiply : Gain  Gain=10  ParamDataTypeStr=Inherit: Same as input  LockScale=on
  Sum : Sum  Inputs=|++
  Out1 : Outport
  wires:
  Bitwise OR1/1 -> Sum/2
  Constant1/1 -> Bitwise OR/2
  Bit Shift/1 -> Multiply/1
  Bitwise OR/1 -> Bit Shift/1
  Data Type Conversion/1 -> Sum/1
  Multiply/1 -> Data Type Conversion/1
  Constant2/1 -> Bitwise OR1/2
  Sum/1 -> Out1/1
  In1/1 -> Bitwise OR1/1, Bitwise OR/1

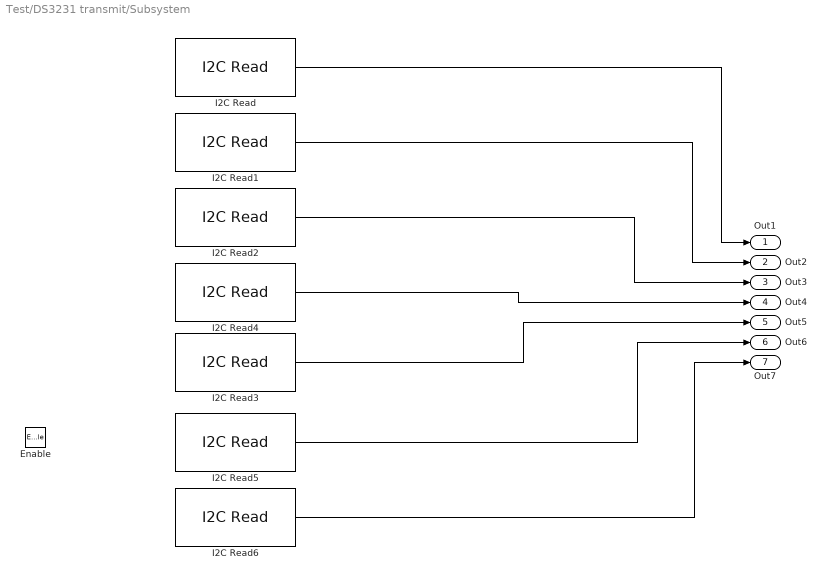
== system Test/DS3231 transmit/Subsystem ==
  Enable : EnablePort
  I2C Read : arduinolib/I2C Read  I2CModule=0  Mode=Master  SlaveAddress=0x68  SlaveByteOrder=BigEndian  Direction=Receiver  RegisterAddressMode=on  RegisterAddress=0x00  SlaveDataType=uint8  DataLength=1  NoAck=off  RepeatedStart=off  OutputStatus=off  blockPlatform=ARDUINO  SampleTime=0.5
  I2C Read1 : arduinolib/I2C Read  I2CModule=0  Mode=Master  SlaveAddress=0x68  SlaveByteOrder=BigEndian  Direction=Receiver  RegisterAddressMode=on  RegisterAddress=0x01  SlaveDataType=uint8  DataLength=1  NoAck=off  RepeatedStart=off  OutputStatus=off  blockPlatform=ARDUINO  SampleTime=0.5
  I2C Read2 : arduinolib/I2C Read  I2CModule=0  Mode=Master  SlaveAddress=0x68  SlaveByteOrder=BigEndian  Direction=Receiver  RegisterAddressMode=on  RegisterAddress=0x02  SlaveDataType=uint8  DataLength=1  NoAck=off  RepeatedStart=off  OutputStatus=off  blockPlatform=ARDUINO  SampleTime=0.5
  I2C Read3 : arduinolib/I2C Read  I2CModule=0  Mode=Master  SlaveAddress=0x68  SlaveByteOrder=BigEndian  Direction=Receiver  RegisterAddressMode=on  RegisterAddress=0x04  SlaveDataType=uint8  DataLength=1  NoAck=off  RepeatedStart=off  OutputStatus=off  blockPlatform=ARDUINO  SampleTime=0.5
  I2C Read4 : arduinolib/I2C Read  I2CModule=0  Mode=Master  SlaveAddress=0x68  SlaveByteOrder=BigEndian  Direction=Receiver  RegisterAddressMode=on  RegisterAddress=0x03  SlaveDataType=uint8  DataLength=1  NoAck=off  RepeatedStart=off  OutputStatus=off  blockPlatform=ARDUINO  SampleTime=0.5
  I2C Read5 : arduinolib/I2C Read  I2CModule=0  Mode=Master  SlaveAddress=0x68  SlaveByteOrder=BigEndian  Direction=Receiver  RegisterAddressMode=on  RegisterAddress=0x05  SlaveDataType=uint8  DataLength=1  NoAck=off  RepeatedStart=off  OutputStatus=off  blockPlatform=ARDUINO  SampleTime=0.5
  I2C Read6 : arduinolib/I2C Read  I2CModule=0  Mode=Master  SlaveAddress=0x68  SlaveByteOrder=BigEndian  Direction=Receiver  RegisterAddressMode=on  RegisterAddress=0x06  SlaveDataType=uint8  DataLength=1  NoAck=off  RepeatedStart=off  OutputStatus=off  blockPlatform=ARDUINO  SampleTime=0.5
  Out1 : Outport
  Out2 : Outport  Port=2
  Out3 : Outport  Port=3
  Out4 : Outport  Port=4
  Out5 : Outport  Port=5
  Out6 : Outport  Port=6
  Out7 : Outport  Port=7
  wires:
  I2C Read4/1 -> Out4/1
  I2C Read1/1 -> Out2/1
  I2C Read/1 -> Out1/1
  I2C Read5/1 -> Out6/1
  I2C Read2/1 -> Out3/1
  I2C Read3/1 -> Out5/1
  I2C Read6/1 -> Out7/1

== system Test/DS3231 transmit/minuteConvert ==
  note: LSB
  note: MSB
  In1 : Inport
  Bit Shift : hdlsllib/Logic and Bit Operations/Bit Shift  mode=Shift Right Logical  N=4
  Bitwise OR : simulink/Logic and Bit Operations/Bitwise Operator  logicop=AND  UseBitMask=off  NumInputPorts=2  BitMask=bin2dec('0000FFFF')  BitMaskRealWorld=Stored Integer
      settings: LibrarySourceBlock=|
      | simulink/Quick Insert/Logic and Bit
      | Operations/Bitwise OR
  Bitwise OR1 : simulink/Logic and Bit Operations/Bitwise Operator  logicop=AND  UseBitMask=off  NumInputPorts=2  BitMask=bin2dec('0000FFFF')  BitMaskRealWorld=Stored Integer
      settings: LibrarySourceBlock=|
      | simulink/Quick Insert/Logic and Bit
      | Operations/Bitwise OR
  Constant1 : Constant  Value=0xF0
  Constant2 : Constant  Value=0x0F
  Data Type Conversion : DataTypeConversion  OutDataTypeStr=uint8  SaturateOnIntegerOverflow=off  RndMeth=Floor
  Multiply : Gain  Gain=10  ParamDataTypeStr=Inherit: Same as input  LockScale=on
  Sum : Sum  Inputs=|++
  Out1 : Outport
  wires:
  Bitwise OR1/1 -> Sum/2
  Constant1/1 -> Bitwise OR/2
  Bit Shift/1 -> Multiply/1
  Bitwise OR/1 -> Bit Shift/1
  Data Type Conversion/1 -> Sum/1
  Multiply/1 -> Data Type Conversion/1
  Constant2/1 -> Bitwise OR1/2
  Sum/1 -> Out1/1
  In1/1 -> Bitwise OR1/1, Bitwise OR/1
